simulink model "getEncoders"  (R2019a)
settings: Solver=FixedStepAuto  StartTime=0.0  StopTime=10.0  FixedStep=Ts  RelTol=1e-3
settings Model: Creator=bspoe  LastModifiedBy=florian

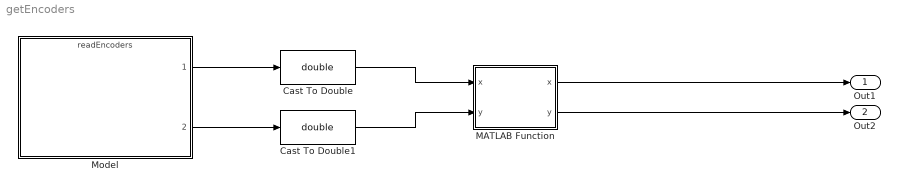
== system getEncoders ==
  Cast To Double : DataTypeConversion  OutDataTypeStr=double
  Cast To Double1 : DataTypeConversion  OutDataTypeStr=double
  MATLAB Function : MATLAB Function  TreatAsAtomicUnit=on
  Model : ModelReference  ModelNameDialog=readEncoders.slx  SimulationMode=Normal  ModelReferenceVersion=1.8
  Out1 : Outport
  Out2 : Outport  Port=2
  wires:
  Model/1 -> Cast To Double/1
  Model/2 -> Cast To Double1/1
  Cast To Double/1 -> MATLAB Function/1("x ")
  Cast To Double1/1 -> MATLAB Function/2("y ")
  MATLAB Function/1(x) -> Out1/1
  MATLAB Function/2(y) -> Out2/1

== matlab function getEncoders/MATLAB Function ==
  data: x output; x input; y output; y input
function [x, y] = fcn(x, y)
%Will depend on the gear ratios used
x = x * 51.45 * 2.88 * 12;
y = y * 51.45 * 2.88 * 12;
